simulink model "FailSafeTimer"  (R2025a)
settings: Solver=VariableStepAuto  StartTime=0.0  StopTime=10.0  RelTol=1e-3
libraries: simulink x2
settings Model: Creator=mahij  LastModifiedBy=mahij

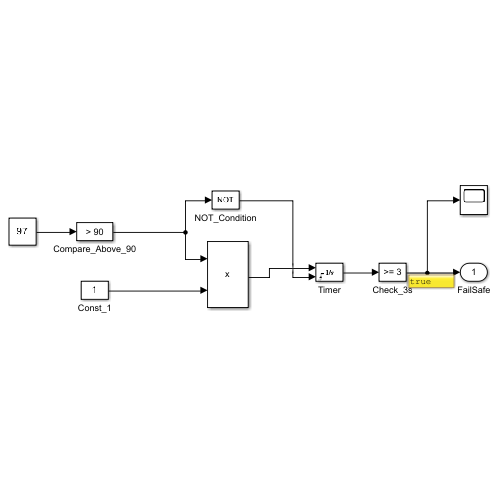
[thumbnail: Simulink's stored preview of the top-level diagram]
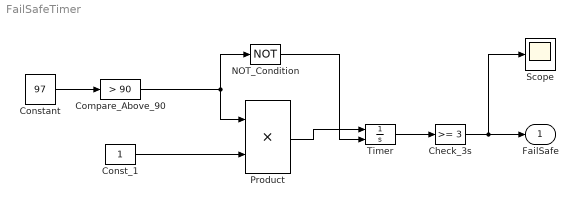
== system FailSafeTimer ==
  Check_3s : simulink/Logic and Bit Operations/Compare To Constant  relop=>=  const=3  OutDataTypeStr=boolean
  Compare_Above_90 : simulink/Logic and Bit Operations/Compare To Constant  relop=>  const=90  OutDataTypeStr=boolean
  Const_1 : Constant
  Constant : Constant  Value=97
  NOT_Condition : Logic  Operator=NOT  AllPortsSameDT=off  OutDataTypeStr=boolean
  Product : Product
  Scope : Scope
  Timer : Integrator  ExternalReset=rising
  FailSafe : Outport
  wires:
  Constant/1 -> Compare_Above_90/1
  Compare_Above_90/1 -> Product/1, NOT_Condition/1
  Const_1/1 -> Product/2
  Product/1 -> Timer/1
  Timer/1 -> Check_3s/1
  Check_3s/1 -> Scope/1, FailSafe/1
  NOT_Condition/1 -> Timer/2
